simulink model "Lab06_tostudents_2020"  (R2020b)
settings: Solver=FixedStepAuto  StartTime=0.0  StopTime=inf  FixedStep=0.01  RelTol=1e-3  EnableMultiTasking=on
InitFcn:
  | Ts = 0.01;
  | IniT = 8;
  | FilterGain = 0.02;
libraries: arduinolib x2
settings Model: SimulationMode=external  SILPILModeSetting=veronly  ExtModeTrigDuration=2  Creator=bnewman  LastModifiedBy=hetia
settings DataIOCC: ReturnWorkspaceOutputs=off
settings OptimizationCC: PassReuseOutputArgsThreshold=0  MaxStackSize=64
settings DebuggingCC: ParameterTunabilityLossMsg=error  PregeneratedLibrarySubsystemCodeDiagnostic=none  ArithmeticOperatorsInVariantConditions=warning
settings HardwareCC: ProdBitPerInt=16  ProdBitPerPointer=16  ProdBitPerSizeT=16  ProdBitPerPtrDiffT=16  ProdLargestAtomicFloat=None  ProdWordSize=8  ProdHWDeviceType=Atmel->AVR
settings SFSimCC: SimUseLocalCustomCode=off  MATLABDynamicMemAlloc=off  CustomCodeUndefinedFunction=UseInterfaceOnly
settings RTWCC: Description=Embedded Coder  SystemTargetFile=ert.tlc  HardwareBoard=Arduino Uno  TemplateMakefile=ert_default_tmf  RTWVerbose=off  RTWUseLocalCustomCode=off  Toolchain=Arduino AVR  BuildConfiguration=Faster Runs
settings CodeAppCC: ForceParamTrailComments=on  OperatorAnnotations=on  MangleLength=10
settings ERTTargetCC: ERTCustomFileBanners=off  SupportContinuousTime=on  SupportNonInlinedSFcns=on  RemoveResetFunc=off  SupportVariableSizeSignals=on  ModelStepFunctionPrototypeControlCompliant=off  ExtMode=on  ExtModeStaticAllocSize=250  ExtModeMexArgs='172.20.10.10' 0 17725  ERTSrcFileBannerTemplate=codertarget_code_template.cgt  ERTHdrFileBannerTemplate=codertarget_code_template.cgt  ERTDataSrcFileTemplate=codertarget_code_template.cgt  ERTDataHdrFileTemplate=codertarget_code_template.cgt

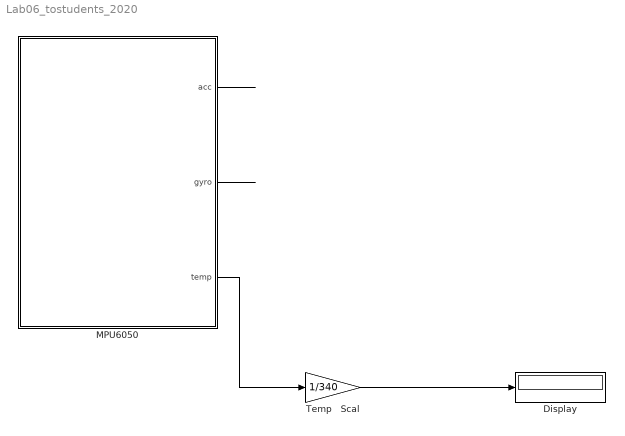
== system Lab06_tostudents_2020 ==
  Display : Display
  MPU6050 : Stateflow chart  TreatAsAtomicUnit=on
  Temp   Scal : Gain  Gain=1/340  OutDataTypeStr=double
  wires:
  MPU6050/2(gyro) -> ?
  MPU6050/1(acc) -> ?
  MPU6050/3(temp) -> Temp   Scal/1
  Temp   Scal/1 -> Display/1

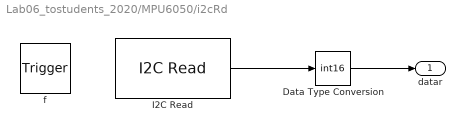
== system Lab06_tostudents_2020/MPU6050/i2cRd ==
  f : TriggerPort  TriggerType=function-call  VariantControl=Variant  SampleTime=-1
      settings: CopyFcn=Stateflow.SLINSF.SimulinkMan.removeBlockPreDeleteFcn  PreDeleteFcn=Stateflow.SLINSF.SimulinkMan.unsafePredeleteFcn
  Data Type Conversion : DataTypeConversion  OutDataTypeStr=int16
  I2C Read : arduinolib/I2C Read  I2CModule=0  Mode=Master  SlaveAddress=hex2dec( '68' )  SlaveByteOrder=BigEndian  Direction=Receiver  RegisterAddressMode=on  RegisterAddress=hex2dec( '3b' )  SlaveDataType=uint16  DataLength=7  NoAck=off  RepeatedStart=off  OutputStatus=off  blockPlatform=arduino  SampleTime=-1
      settings: SourceProductBaseCode=ARDUINO
  datar : Outport  OutDataTypeStr=int16  Unit=1  PortDimensions=7  VectorParamsAs1DForOutWhenUnconnected=off
  wires:
  I2C Read/1 -> Data Type Conversion/1
  Data Type Conversion/1 -> datar/1

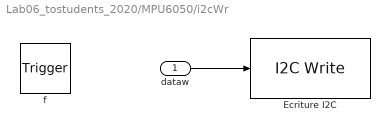
== system Lab06_tostudents_2020/MPU6050/i2cWr ==
  dataw : Inport  OutDataTypeStr=uint16  Unit=1  PortDimensions=1
  f : TriggerPort  TriggerType=function-call  VariantControl=Variant  SampleTime=-1
      settings: CopyFcn=Stateflow.SLINSF.SimulinkMan.removeBlockPreDeleteFcn  PreDeleteFcn=Stateflow.SLINSF.SimulinkMan.unsafePredeleteFcn
  Ecriture I2C : arduinolib/I2C Write  Priority=1  I2CModule=0  Mode=Master  SlaveAddress=hex2dec( '68' )  SlaveByteOrder=BigEndian  Direction=Transmitter  RegisterAddressMode=on  RegisterAddress=hex2dec( '6B' )  SlaveDataType=uint16  DataLength=1  NoAck=off  RepeatedStart=off  OutputStatus=off  blockPlatform=arduino
      settings: SourceProductBaseCode=ARDUINO
  wires:
  dataw/1 -> Ecriture I2C/1

== stateflow chart Lab06_tostudents_2020/MPU6050 ==
  state initialisation
    en:
    i2cWr(uint16(hex2dec( '6B00' )));%Power on
    i2cWr(uint16(hex2dec( '1B10' )));%gyro 0x10=1000°/s
    i2cWr(uint16(hex2dec( '1C08' )));%acce 0x08= 4G
    i2cWr(uint16(hex2dec( '1A06' )));%filtrage+actu 0x06= 19ms
    i2cWr(uint16(hex2dec( '3710' )));%INT_PIN_CFG
    i2cWr(uint16(hex2dec( '3800' )));%Interrupt Enable 0 désactivé
  state i2cWr(dataw) [function]
  state datar = i2cRd [function]
  state Lecture_acceleration3_axes
    during:
    i2cWr(uint16(hex2dec( '1C08' )));%acce 0x08= 4G
    i2cWr(uint16(hex2dec( '3800' )));%Interrupt Enable 0 désactivé
    val=i2cRd;
    acc=val(1:3);
    gyro=val(5:7);
    temp=val(4:4);
  (default) -> initialisation
  initialisation -> Lecture_acceleration3_axes
  data: dataw function_input uint16 size=1; datar function_output int16 size=7; acc output int16 size=3; gyro output int16 size=3; val local int16 size=7; temp output int16 size=1
